simulink model "q3_d"  (R2016a)
settings: Solver=ode3  StartTime=0.0  StopTime=50  FixedStep=0.001  RelTol=1e-3
settings Model: Creator=Ahmet Asım  LastModifiedBy=Ahmet Asım

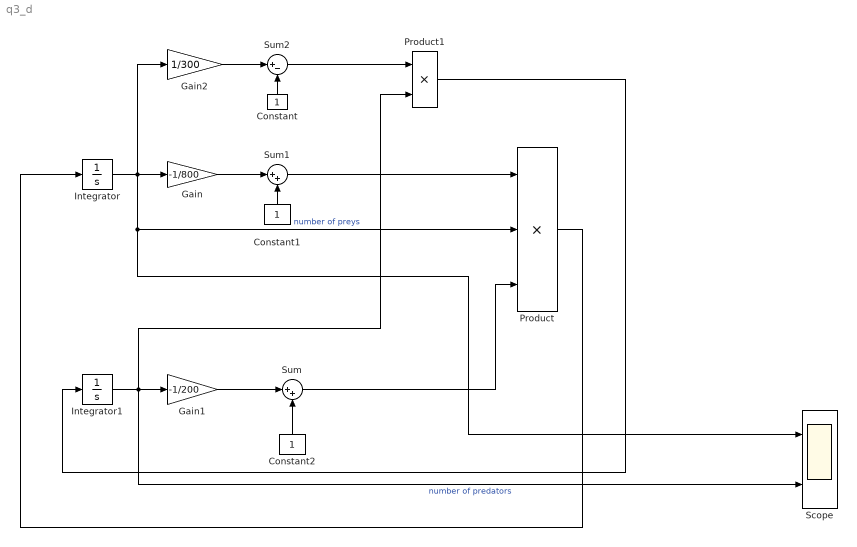
== system q3_d ==
  Constant : Constant
  Constant1 : Constant
  Constant2 : Constant
  Gain : Gain  Gain=-1/800
  Gain1 : Gain  Gain=-1/200
  Gain2 : Gain  Gain=1/300
  Integrator : Integrator  InitialCondition=400
  Integrator1 : Integrator  InitialCondition=100
  Product : Product  Inputs=3
  Product1 : Product
  Scope : Scope  NumInputPorts=2
  Sum : Sum  Inputs=|++
  Sum1 : Sum  Inputs=|++
  Sum2 : Sum  Inputs=|+-
  wires:
  Integrator/1 -> Gain2/1, Scope/1, Product/2, Gain/1  "number of preys"
  Constant/1 -> Sum2/2
  Constant1/1 -> Sum1/2
  Constant2/1 -> Sum/2
  Sum2/1 -> Product1/1
  Gain/1 -> Sum1/1
  Sum1/1 -> Product/1
  Integrator1/1 -> Scope/2, Product1/2, Gain1/1  "number of predators"
  Gain1/1 -> Sum/1
  Sum/1 -> Product/3
  Gain2/1 -> Sum2/1
  Product1/1 -> Integrator1/1
  Product/1 -> Integrator/1
